simulink model "simulacao_figs_capacitorres"  (R2014a)
settings: Solver=ode45  StartTime=0.0  StopTime=0.01  RelTol=1e-3
libraries: powerlib x33
settings Model: Creator=Joao  LastModifiedBy=Joao

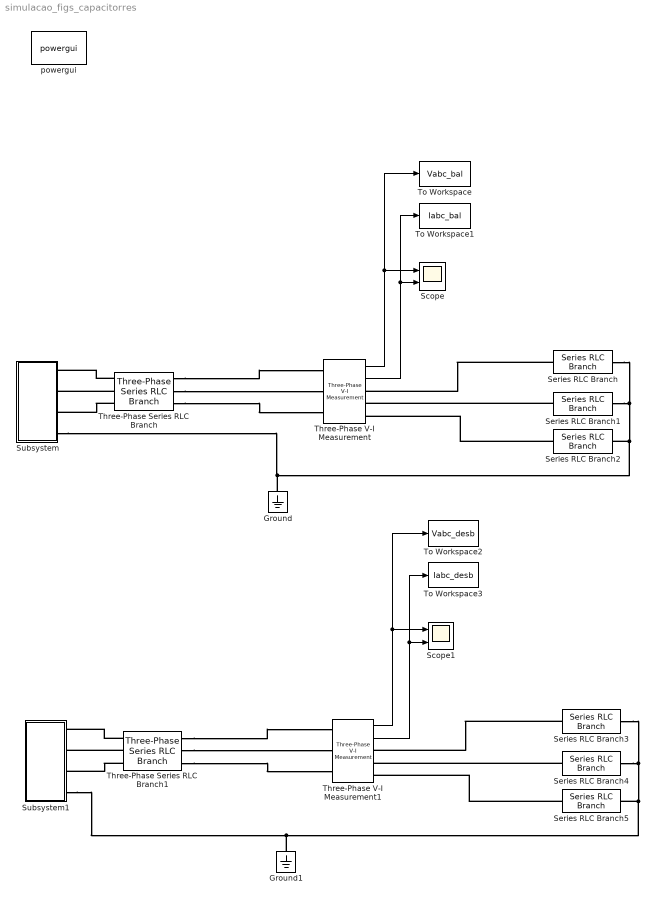
== system simulacao_figs_capacitorres ==
  Ground : powerlib/Elements/Ground  LConnTagsString=a
  Ground1 : powerlib/Elements/Ground  LConnTagsString=a
  Scope : Scope  NumInputPorts=2
      settings: YMin=-250~-17.5  YMax=250~17.5
  Scope1 : Scope  NumInputPorts=2
      settings: YMin=-250~-17.5  YMax=250~17.5
  Series RLC Branch{,1..2,4..5} (5 alike) : powerlib/Elements/Series RLC Branch  LConnTagsString=__new0  RConnTagsString=__new0  BranchType=C  Resistance=1  Inductance=1e-3  SetiL0=off  InitialCurrent=0  Capacitance=10e-6  Setx0=off  InitialVoltage=0  Measurements=None
  Series RLC Branch3 : powerlib/Elements/Series RLC Branch  LConnTagsString=__new0  RConnTagsString=__new0  BranchType=C  Resistance=1  Inductance=1e-3  SetiL0=off  InitialCurrent=0  Capacitance=30e-6  Setx0=off  InitialVoltage=0  Measurements=None
  Subsystem : Subsystem  mask{Vp=115*sqrt(2), Vn=0, phin=0, Vz=0, phi0=0, f=400}
      mask prompts: Vp "Tensão Sequência Positiva"; Vn "Tensão Sequência Negativa"; phin "Defasagem Sequência Negativa"; Vz "Tensão Sequência Zero"; phi0 "Defasagem Sequência Zero"; f "Frequência"
  Subsystem1 : Subsystem  mask{Vp=115*sqrt(2), Vn=0, phin=0, Vz=0, phi0=0, f=400}
      mask prompts: Vp "Tensão Sequência Positiva"; Vn "Tensão Sequência Negativa"; phin "Defasagem Sequência Negativa"; Vz "Tensão Sequência Zero"; phi0 "Defasagem Sequência Zero"; f "Frequência"
  Three-Phase Series RLC Branch : powerlib/Elements/Three-Phase Series RLC Branch  LConnTagsString=A|B|C  RConnTagsString=A|B|C  BranchType=R  Resistance=1  Inductance=eps  Capacitance=1e-6  Measurements=None
  Three-Phase Series RLC Branch1 : powerlib/Elements/Three-Phase Series RLC Branch  LConnTagsString=A|B|C  RConnTagsString=A|B|C  BranchType=R  Resistance=1  Inductance=eps  Capacitance=1e-6  Measurements=None
  Three-Phase V-I Measurement : powerlib/Measurements/Three-Phase V-I Measurement  VoltageMeasurement=phase-to-ground  SetLabelV=off  LabelV=Vabc  Vpu=off  VpuLL=off  CurrentMeasurement=yes  SetLabelI=off  LabelI=Iabc  Ipu=off  Pbase=100e6  Vbase=500e3  OutputType=Complex  PhasorSimulation=off  PSBequivalent=0
  Three-Phase V-I Measurement1 : powerlib/Measurements/Three-Phase V-I Measurement  VoltageMeasurement=phase-to-ground  SetLabelV=off  LabelV=Vabc  Vpu=off  VpuLL=off  CurrentMeasurement=yes  SetLabelI=off  LabelI=Iabc  Ipu=off  Pbase=100e6  Vbase=500e3  OutputType=Complex  PhasorSimulation=off  PSBequivalent=0
  To Workspace : ToWorkspace  VariableName=Vabc_bal  SaveFormat=Structure With Time  SampleTime=-1
  To Workspace1 : ToWorkspace  VariableName=Iabc_bal  SaveFormat=Structure With Time  SampleTime=-1
  To Workspace2 : ToWorkspace  VariableName=Vabc_desb  SaveFormat=Structure With Time  SampleTime=-1
  To Workspace3 : ToWorkspace  VariableName=Iabc_desb  SaveFormat=Structure With Time  SampleTime=-1
  powergui : powerlib/powergui  Priority=1  SimulationMode=Discrete  SolverType=Tustin  SampleTime=1e-7  frequency=60  SPID=off  DisableSnubberDevices=off  DisableRonSwitches=off  DisableVfSwitches=off  SwTol=0  Interpol=off  DisplayEquations=off  Ts=100  methode=off  frequencyindice=400  Pbase=100e6  ErrMax=1e-4  Iterations=50  UnitsV=kV  UnitsW=MW  FunctionMessages=off  echomessages=off  HookPort=off  EnableUseOfTLC=off  x0status=blocks  RestoreLinks=warning  ResistiveCurrentMeasurement=off  Frange=[0:2:500]  Ylog=off  Xlog=on  ShowGrid=off  save=off  variable=ZData  structure=0  ZoomFFT=off  StartTime=0.0  cycles=1  DisplayStyle=1  fundamental=60  FreqAxis=off  MaxFrequency=1000  frequencyindicesteady=1  RmsSteady=1  display=off
  wires:
  Three-Phase V-I Measurement/1 -> Scope/1, To Workspace/1
  Three-Phase V-I Measurement/2 -> Scope/2, To Workspace1/1
  Three-Phase V-I Measurement1/1 -> Scope1/1, To Workspace2/1
  Three-Phase V-I Measurement1/2 -> Scope1/2, To Workspace3/1
  connections:
  Three-Phase Series RLC Branch/RConn2 -- Three-Phase V-I Measurement/LConn2
  Series RLC Branch/LConn1 -- Three-Phase V-I Measurement/RConn1
  Series RLC Branch1/LConn1 -- Three-Phase V-I Measurement/RConn2
  Series RLC Branch2/LConn1 -- Three-Phase V-I Measurement/RConn3
  Subsystem/RConn4 -- Ground/LConn1 -- Series RLC Branch/RConn1 -- Series RLC Branch1/RConn1 -- Series RLC Branch2/RConn1
  Three-Phase Series RLC Branch/LConn2 -- Subsystem/RConn2
  Three-Phase Series RLC Branch/RConn1 -- Three-Phase V-I Measurement/LConn1
  Three-Phase Series RLC Branch/RConn3 -- Three-Phase V-I Measurement/LConn3
  Three-Phase Series RLC Branch/LConn1 -- Subsystem/RConn1
  Three-Phase Series RLC Branch/LConn3 -- Subsystem/RConn3
  Series RLC Branch4/RConn1 -- Series RLC Branch3/RConn1 -- Ground1/LConn1 -- Subsystem1/RConn4 -- Series RLC Branch5/RConn1
  Series RLC Branch5/LConn1 -- Three-Phase V-I Measurement1/RConn3
  Series RLC Branch4/LConn1 -- Three-Phase V-I Measurement1/RConn2
  Three-Phase Series RLC Branch1/LConn3 -- Subsystem1/RConn3
  Three-Phase Series RLC Branch1/RConn3 -- Three-Phase V-I Measurement1/LConn3
  Three-Phase Series RLC Branch1/RConn1 -- Three-Phase V-I Measurement1/LConn1
  Three-Phase Series RLC Branch1/LConn1 -- Subsystem1/RConn1
  Three-Phase Series RLC Branch1/LConn2 -- Subsystem1/RConn2
  Series RLC Branch3/LConn1 -- Three-Phase V-I Measurement1/RConn1
  Three-Phase Series RLC Branch1/RConn2 -- Three-Phase V-I Measurement1/LConn2

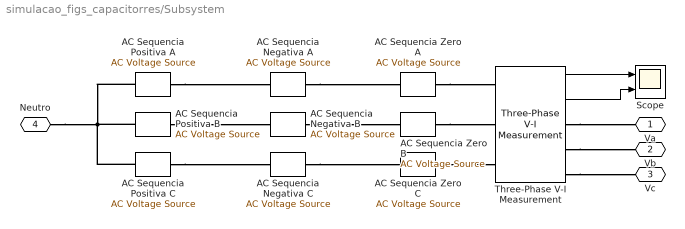
== system simulacao_figs_capacitorres/Subsystem ==
  AC Sequencia Negativa A : powerlib/Electrical Sources/AC Voltage Source  Amplitude=Vn  Phase=0+phin  Frequency=f  SampleTime=0  Measurements=None
  AC Sequencia Negativa B : powerlib/Electrical Sources/AC Voltage Source  Amplitude=Vn  Phase=120+phin  Frequency=f  SampleTime=0  Measurements=None
  AC Sequencia Negativa C : powerlib/Electrical Sources/AC Voltage Source  Amplitude=Vn  Phase=-120+phin  Frequency=f  SampleTime=0  Measurements=None
  AC Sequencia Positiva A : powerlib/Electrical Sources/AC Voltage Source  Amplitude=Vp  Phase=0  Frequency=f  SampleTime=0  Measurements=None
  AC Sequencia Positiva B : powerlib/Electrical Sources/AC Voltage Source  Amplitude=Vp  Phase=-120  Frequency=f  SampleTime=0  Measurements=None
  AC Sequencia Positiva C : powerlib/Electrical Sources/AC Voltage Source  Amplitude=Vp  Phase=+120  Frequency=f  SampleTime=0  Measurements=None
  AC Sequencia Zero A : powerlib/Electrical Sources/AC Voltage Source  Amplitude=Vz  Phase=0+phi0  Frequency=f  SampleTime=0  Measurements=None
  AC Sequencia Zero B : powerlib/Electrical Sources/AC Voltage Source  Amplitude=Vz  Phase=0+phi0  Frequency=f  SampleTime=0  Measurements=None
  AC Sequencia Zero C : powerlib/Electrical Sources/AC Voltage Source  Amplitude=Vz  Phase=0+phi0  Frequency=f  SampleTime=0  Measurements=None
  Scope : Scope  NumInputPorts=2
      settings: YMin=-6~-0.8  YMax=6~0.8  SaveName=ScopeData14
  Three-Phase V-I Measurement : powerlib/Measurements/Three-Phase V-I Measurement  VoltageMeasurement=phase-to-ground  SetLabelV=off  LabelV=Vabc  Vpu=off  VpuLL=off  CurrentMeasurement=yes  SetLabelI=off  LabelI=Iabc  Ipu=off  Pbase=100e6  Vbase=500e3  OutputType=Complex  PhasorSimulation=off  PSBequivalent=0
  Va : PMIOPort  Port=1  Side=Right
  Vb : PMIOPort  Port=2  Side=Right
  Vc : PMIOPort  Port=3  Side=Right
  Neutro : PMIOPort  Port=4  Side=Right
  wires:
  Three-Phase V-I Measurement/2 -> Scope/2
  Three-Phase V-I Measurement/1 -> Scope/1
  connections:
  Three-Phase V-I Measurement/RConn3 -- Vc/RConn1
  Three-Phase V-I Measurement/RConn2 -- Vb/RConn1
  Three-Phase V-I Measurement/RConn1 -- Va/RConn1
  AC Sequencia Zero C/RConn1 -- Three-Phase V-I Measurement/LConn3
  AC Sequencia Zero B/RConn1 -- Three-Phase V-I Measurement/LConn2
  AC Sequencia Zero A/RConn1 -- Three-Phase V-I Measurement/LConn1
  AC Sequencia Negativa C/RConn1 -- AC Sequencia Zero C/LConn1
  AC Sequencia Negativa B/RConn1 -- AC Sequencia Zero B/LConn1
  AC Sequencia Negativa A/RConn1 -- AC Sequencia Zero A/LConn1
  AC Sequencia Positiva A/RConn1 -- AC Sequencia Negativa A/LConn1
  AC Sequencia Positiva B/RConn1 -- AC Sequencia Negativa B/LConn1
  AC Sequencia Positiva C/RConn1 -- AC Sequencia Negativa C/LConn1
  AC Sequencia Positiva B/LConn1 -- AC Sequencia Positiva C/LConn1 -- Neutro/RConn1 -- AC Sequencia Positiva A/LConn1

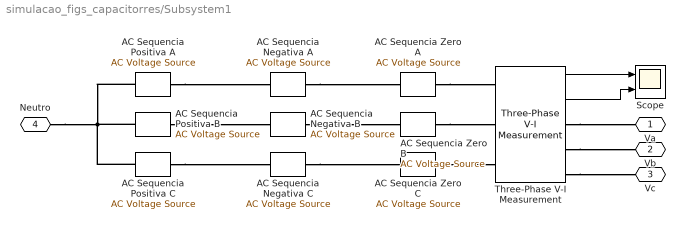
== system simulacao_figs_capacitorres/Subsystem1 ==
  AC Sequencia Negativa A : powerlib/Electrical Sources/AC Voltage Source  Amplitude=Vn  Phase=0+phin  Frequency=f  SampleTime=0  Measurements=None
  AC Sequencia Negativa B : powerlib/Electrical Sources/AC Voltage Source  Amplitude=Vn  Phase=120+phin  Frequency=f  SampleTime=0  Measurements=None
  AC Sequencia Negativa C : powerlib/Electrical Sources/AC Voltage Source  Amplitude=Vn  Phase=-120+phin  Frequency=f  SampleTime=0  Measurements=None
  AC Sequencia Positiva A : powerlib/Electrical Sources/AC Voltage Source  Amplitude=Vp  Phase=0  Frequency=f  SampleTime=0  Measurements=None
  AC Sequencia Positiva B : powerlib/Electrical Sources/AC Voltage Source  Amplitude=Vp  Phase=-120  Frequency=f  SampleTime=0  Measurements=None
  AC Sequencia Positiva C : powerlib/Electrical Sources/AC Voltage Source  Amplitude=Vp  Phase=+120  Frequency=f  SampleTime=0  Measurements=None
  AC Sequencia Zero A : powerlib/Electrical Sources/AC Voltage Source  Amplitude=Vz  Phase=0+phi0  Frequency=f  SampleTime=0  Measurements=None
  AC Sequencia Zero B : powerlib/Electrical Sources/AC Voltage Source  Amplitude=Vz  Phase=0+phi0  Frequency=f  SampleTime=0  Measurements=None
  AC Sequencia Zero C : powerlib/Electrical Sources/AC Voltage Source  Amplitude=Vz  Phase=0+phi0  Frequency=f  SampleTime=0  Measurements=None
  Scope : Scope  NumInputPorts=2
      settings: YMin=-6~-0.8  YMax=6~0.8  SaveName=ScopeData14
  Three-Phase V-I Measurement : powerlib/Measurements/Three-Phase V-I Measurement  VoltageMeasurement=phase-to-ground  SetLabelV=off  LabelV=Vabc  Vpu=off  VpuLL=off  CurrentMeasurement=yes  SetLabelI=off  LabelI=Iabc  Ipu=off  Pbase=100e6  Vbase=500e3  OutputType=Complex  PhasorSimulation=off  PSBequivalent=0
  Va : PMIOPort  Port=1  Side=Right
  Vb : PMIOPort  Port=2  Side=Right
  Vc : PMIOPort  Port=3  Side=Right
  Neutro : PMIOPort  Port=4  Side=Right
  wires:
  Three-Phase V-I Measurement/2 -> Scope/2
  Three-Phase V-I Measurement/1 -> Scope/1
  connections:
  Three-Phase V-I Measurement/RConn3 -- Vc/RConn1
  Three-Phase V-I Measurement/RConn2 -- Vb/RConn1
  Three-Phase V-I Measurement/RConn1 -- Va/RConn1
  AC Sequencia Zero C/RConn1 -- Three-Phase V-I Measurement/LConn3
  AC Sequencia Zero B/RConn1 -- Three-Phase V-I Measurement/LConn2
  AC Sequencia Zero A/RConn1 -- Three-Phase V-I Measurement/LConn1
  AC Sequencia Negativa C/RConn1 -- AC Sequencia Zero C/LConn1
  AC Sequencia Negativa B/RConn1 -- AC Sequencia Zero B/LConn1
  AC Sequencia Negativa A/RConn1 -- AC Sequencia Zero A/LConn1
  AC Sequencia Positiva A/RConn1 -- AC Sequencia Negativa A/LConn1
  AC Sequencia Positiva B/RConn1 -- AC Sequencia Negativa B/LConn1
  AC Sequencia Positiva C/RConn1 -- AC Sequencia Negativa C/LConn1
  AC Sequencia Positiva B/LConn1 -- AC Sequencia Positiva C/LConn1 -- Neutro/RConn1 -- AC Sequencia Positiva A/LConn1
